simulink model "Model"  (R2023a)
settings: Solver=ode3  StartTime=0.0  StopTime=2.0  FixedStep=0.0001  RelTol=1e-3
values from neighbouring files (symbols this model uses):
  J2 = 1.26e-3    (= 0.00126)    [system_init.m]
libraries: neural x24
(part 1 of 2)
settings Model: SimulationMode=accelerator  Creator=04  LastModifiedBy=23688
settings SolverCC: AlgebraicLoopSolver=TrustRegion
settings DataIOCC: ReturnWorkspaceOutputs=off
settings DebuggingCC: UnconnectedInputMsg=warning  UnconnectedOutputMsg=warning  UnconnectedLineMsg=warning
settings ModelReferenceCC: EnableRefExpFcnMdlSchedulingChecks=on
settings RTWCC: DLArmComputeVersion=19.05

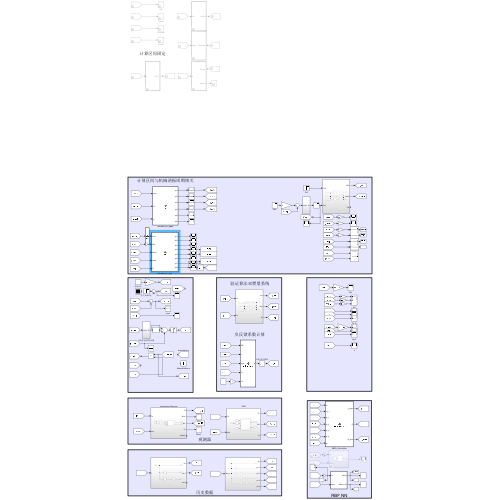
[thumbnail: Simulink's stored preview of the top-level diagram]
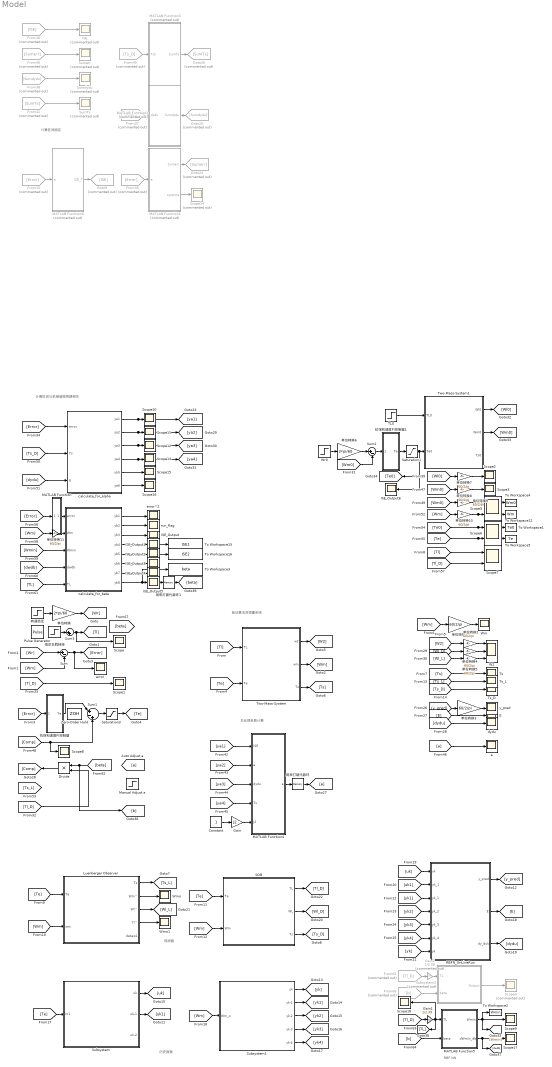
== system Model ==
  note: 观测器
  note: 历史数据
  note: 计算区间固定
  note: 计算区间与机械谐振周期相关
  note: 验证算法双惯量系统
  note: 负反馈系数计算
  note: RBF NN
  " Luenberger Observer" : Subsystem
  Constant : Constant
  Divide : Product  Inputs=**
  E : Scope
  From15 : From  Commented=on  GotoTag=Error
  From16 : From  Commented=on  GotoTag=ISE
  From35 : From  Commented=on  GotoTag=Error
  From36 : From  Commented=on  GotoTag=Sumerr
  From37 : From  Commented=on  GotoTag=dydu
  From38 : From  Commented=on  GotoTag=Sumdydu
  From40 : From  Commented=on  GotoTag=Ts_D
  From41 : From  Commented=on  GotoTag=SumTs
  From65 : From  Commented=on  GotoTag=Tl_D
  From66 : From  Commented=on  GotoTag=b
  Gain : Gain  Gain=J2
  Gain1 : Gain  Gain=1/2.39
  Gain2 : Gain  Commented=on  Gain=1/2.39
  Goto24 : Goto  Commented=on  GotoTag=Sumerr
  Goto25 : Goto  Commented=on  GotoTag=Sumdydu
  Goto26 : Goto  Commented=on  GotoTag=SumTs
  Goto9 : Goto  Commented=on  GotoTag=ISE
  ISE : Scope  Commented=on
  ISE_Output{,1..6} (7 alike) : Scope
  MATLAB Function : MATLAB Function  TreatAsAtomicUnit=on
  MATLAB Function1 : MATLAB Function  Commented=on  TreatAsAtomicUnit=on
  MATLAB Function2 : MATLAB Function  Commented=on  TreatAsAtomicUnit=on
  MATLAB Function3 : MATLAB Function  Commented=on  TreatAsAtomicUnit=on
  MATLAB Function4 : MATLAB Function  TreatAsAtomicUnit=on
  MATLAB Function5 : MATLAB Function  TreatAsAtomicUnit=on
  MATLAB Function6 : MATLAB Function  Commented=on  TreatAsAtomicUnit=on
  Manual Adjust a : Step  Time=0.1  After=0.0  SampleTime=0
  Pulse Generator : DiscretePulseGenerator  PulseType=Time based  Amplitude=2.39*0.7  Period=1  PulseWidth=50  PhaseDelay=1
  RBFN_OnLineRun : MATLAB Function  TreatAsAtomicUnit=on
  SOB : Subsystem
  Saturation1 : Saturate  UpperLimit=2.39*3  LowerLimit=-2.39*3
  Saturation3 : Saturate  UpperLimit=2.39*3  LowerLimit=-2.39*3
  Scope{,1..3,8..13,15..18} (14 alike) : Scope
  Scope14 : Scope  Commented=on
  Scope4 : Scope  Commented=on
  Scope5 : Scope  NumInputPorts=2
  Scope6 : Scope  NumInputPorts=2
  Scope7 : Scope  NumInputPorts=2
  Subsystem : Subsystem
  Subsystem1 : Subsystem
  Subsystem2 : Subsystem  Commented=on
  Sum : Sum  Inputs=|+-
  Sum1 : Sum  Inputs=|+-+
  Sum2 : Sum  Inputs=|+-
  Sum3 : Sum  Inputs=|++
  SumTs : Scope  Commented=on
  Sumdydu : Scope  Commented=on
  Sumerr : Scope  Commented=on
  TL0 : Step  After=2.39*0.5  SampleTime=0
  To Workspace1 : ToWorkspace  VariableName=Te0  SampleTime=-1
  To Workspace12 : ToWorkspace  VariableName=Wm  SampleTime=-1
  To Workspace15 : ToWorkspace  VariableName=ISE1  SampleTime=-1
  To Workspace16 : ToWorkspace  VariableName=ISE2  SampleTime=-1
  To Workspace2 : ToWorkspace  VariableName=Wmin  SampleTime=-1
  To Workspace3 : ToWorkspace  VariableName=beta  SampleTime=-1
  To Workspace4 : ToWorkspace  VariableName=Wm0  SampleTime=-1
  To Workspace5 : ToWorkspace  VariableName=Te  SampleTime=-1
  Ts : Scope
  Ts_D : Scope
  Ts_L : Scope
  Two-Mass-System : Subsystem
  Two-Mass-System1 : Subsystem
  W2 : Scope  NumInputPorts=3
  Wm : Scope
  Wmo : Scope
  Wmo1 : Scope
  Wr0 : Step  Time=0.1  After=1000  SampleTime=0
  Zero-Order Hold : ZeroOrderHold  SampleTime=0.0005
  a : Scope
  calculate_for_alpha : MATLAB Function  TreatAsAtomicUnit=on
  calculate_for_beta : MATLAB Function  TreatAsAtomicUnit=on
  dydu : Scope
  error : Scope
  error^2 : Scope
  run_flag : Scope
  y_pred : Scope
  单位转换 : Gain  Gain=2*pi/60
  单位转换{1..5,7..11} (10 alike) : Gain  Gain=60/2/pi
  单位转换6 : Gain  Gain=2*pi/60
  恒定负载转矩 : Step  After=2.39*0.5  SampleTime=0
  抗饱和速度PI控制器 : Subsystem
  抗饱和速度PI控制器1 : Subsystem
  用来打破代数环 : Memory  InheritSampleTime=on
  用来打破代数环1 : Memory  InheritSampleTime=on
  转速给定 : Step  Time=0.1  After=1000  SampleTime=0
  wires:
  [Tl] -> Two-Mass-System/1(TL)
  Two-Mass-System/2(wm) -> [Wm]
  [Wr] -> Sum/1
  [Wm] -> Sum/2
  Sum/1 -> error/1, [Error]
  [Error] -> 抗饱和速度PI控制器/1(error)
  Two-Mass-System/1(w2) -> [W2]
  Two-Mass-System/3(Ts) -> [Ts]
  [Ts] -> Ts/1
  单位转换/1 -> [Wr]
  [Wm] -> 单位转换1/1
  [Te] -> " Luenberger Observer"/1(Te)
  [Wm] -> " Luenberger Observer"/2(wm)
  [Te] -> SOB/1(Te)
  [Wm] -> SOB/2(Wm)
  " Luenberger Observer"/1(Ts) -> [Ts_L]
  SOB/3(Ts) -> [Ts_D]
  [Ts_L] -> Ts_L/1
  [Ts_D] -> Ts_D/1
  [W2] -> 单位转换2/1
  单位转换2/1 -> W2/1
  [Te] -> Subsystem/1(In1)
  Subsystem/1(uk) -> [uk]
  Subsystem/2(uk-1) -> [uk1]
  Subsystem1/1(yk) -> [yk]
  Subsystem1/2(yk-1) -> [yk1]
  Subsystem1/3(yk-2) -> [yk2]
  Subsystem1/4(yk-3) -> [yk3]
  Subsystem1/5(yk-4) -> [yk4]
  [uk] -> RBFN_OnLineRun/1(uk)
  [uk1] -> RBFN_OnLineRun/2(uk_1)
  [yk] -> RBFN_OnLineRun/7(yk)
  [yk1] -> RBFN_OnLineRun/3(yk_1)
  [yk2] -> RBFN_OnLineRun/4(yk_2)
  [yk3] -> RBFN_OnLineRun/5(yk_3)
  [yk4] -> RBFN_OnLineRun/6(yk_4)
  RBFN_OnLineRun/1(y_pred) -> [y_pred]
  RBFN_OnLineRun/2(E) -> [E]
  [E] -> E/1
  [dydu] -> dydu/1
  SOB/2(WL) -> [Wl_D]
  " Luenberger Observer"/3(Wl^) -> [Wl_L]
  单位转换4/1 -> W2/2
  [Wl_D] -> 单位转换4/1
  单位转换5/1 -> W2/3
  [Wl_L] -> 单位转换5/1
  单位转换1/1 -> Wm/1
  From35/1 -> MATLAB Function1/1(e)
  MATLAB Function1/1(Sumerr) -> Goto24/1
  From16/1 -> ISE/1
  From36/1 -> Sumerr/1
  From37/1 -> MATLAB Function2/1(dydu)
  MATLAB Function2/1(Sumdydu) -> Goto25/1
  From38/1 -> Sumdydu/1
  From40/1 -> MATLAB Function3/1(Tsk)
  MATLAB Function3/1(SumTs) -> Goto26/1
  From41/1 -> SumTs/1
  [ya1] -> MATLAB Function4/1(ISE)
  [ya2] -> MATLAB Function4/2(e)
  [ya3] -> MATLAB Function4/3(dydu)
  [ya4] -> MATLAB Function4/4(Ts)
  [a] -> a/1
  Divide/1 -> [Comp]
  [Te] -> Two-Mass-System/2(Te)
  MATLAB Function6/1(ISE_T) -> Goto9/1
  From15/1 -> MATLAB Function6/1(e)
  Gain/1 -> MATLAB Function4/5(J2)
  Constant/1 -> Gain/1
  SOB/1(TL) -> [Tl_D]
  [Tl_D] -> Scope1/1
  calculate_for_alpha/1(ya1) -> Scope10/1, [ya1]
  calculate_for_alpha/2(ya2) -> Scope11/1, [ya2]
  [Ts_D] -> calculate_for_alpha/2(Ts)
  calculate_for_alpha/3(ya3) -> [ya3], Scope12/1
  [dydu] -> calculate_for_alpha/3(g)
  calculate_for_alpha/4(ya4) -> [ya4], Scope13/1
  MATLAB Function4/1(a) -> 用来打破代数环/1
  RBFN_OnLineRun/3(dy_duk) -> [dydu]
  用来打破代数环/1 -> [a]
  MATLAB Function1/2(systime) -> Scope14/1
  calculate_for_alpha/5(ya5) -> Scope15/1
  calculate_for_alpha/6(ya6) -> Scope16/1
  Saturation3/1 -> [Te]
  " Luenberger Observer"/2(Wm^) -> Wmo/1
  转速给定/1 -> 单位转换/1
  [y_pred] -> 单位转换3/1
  单位转换3/1 -> y_pred/1
  [Wm] -> Subsystem1/1(Wm_o)
  [Error] -> calculate_for_alpha/1(error)
  Sum1/1 -> Saturation3/1
  Sum3/1 -> Scope/1, [Tl]
  calculate_for_beta/1(yb1) -> error^2/1
  calculate_for_beta/2(yb2) -> run_flag/1
  calculate_for_beta/3(yb3) -> ISE_Output/1
  calculate_for_beta/6(yb6) -> ISE_Output3/1
  calculate_for_beta/7(yb7) -> ISE_Output4/1
  [Tl_D] -> Divide/2
  [Error] -> MATLAB Function/1(error)
  抗饱和速度PI控制器/1(Te) -> Sum1/1
  [Comp] -> Scope8/1, Sum1/3
  " Luenberger Observer"/4(Tl^) -> Wmo1/1
  恒定负载转矩/1 -> Sum3/1
  抗饱和速度PI控制器1/1(Te) -> Saturation1/1
  Saturation1/1 -> ISE_Output6/1, [Te0], Two-Mass-System1/2(Te0)
  Wr0/1 -> 单位转换6/1
  Two-Mass-System1/1(Wl0) -> [Wl0]
  Two-Mass-System1/2(Wm0) -> [Wm0]
  单位转换6/1 -> Sum2/1
  Sum2/1 -> 抗饱和速度PI控制器1/1(error)
  [Wm0] -> Sum2/2
  [Wl0] -> 单位转换7/1
  [Wm0] -> 单位转换8/1
  单位转换7/1 -> Scope2/1
  单位转换8/1 -> Scope3/1
  TL0/1 -> Two-Mass-System1/1(TL0)
  [Wm0] -> 单位转换9/1
  单位转换9/1 -> To Workspace4/1, Scope5/1
  单位转换10/1 -> To Workspace12/1, Scope5/2
  [Wm] -> 单位转换10/1
  [Te] -> To Workspace5/1, Scope6/2
  [Tl] -> Scope7/1
  [Tl_D] -> Scope7/2
  MATLAB Function/1(error_output) -> calculate_for_beta/1(error)
  From65/1 -> Gain2/1
  Gain2/1 -> Subsystem2/1(TL)
  From66/1 -> Subsystem2/2(beta)
  Subsystem2/1(Output) -> Scope4/1
  [b] -> MATLAB Function5/2(beta)
  Gain1/1 -> Scope18/1, [TL], MATLAB Function5/1(TL)
  [Tl_D] -> Gain1/1
  MATLAB Function5/1(Wmin) -> To Workspace2/1, [Wmin], Scope9/1
  MATLAB Function5/2(dWmin_db) -> [dwdb], Scope17/1
  calculate_for_beta/5(yb5) -> To Workspace16/1, ISE_Output2/1
  calculate_for_beta/4(yb4) -> To Workspace15/1, ISE_Output1/1
  单位转换11/1 -> calculate_for_beta/2(Wm)
  [Wm] -> 单位转换11/1
  [Wmin] -> calculate_for_beta/3(Wmin)
  [dwdb] -> calculate_for_beta/4(dwdb)
  calculate_for_beta/8(yb8) -> To Workspace3/1, 用来打破代数环1/1, ISE_Output5/1
  [TL] -> calculate_for_beta/5(TL)
  用来打破代数环1/1 -> [beta]
  [beta] -> [b], Divide/1
  [Te0] -> To Workspace1/1, Scope6/1

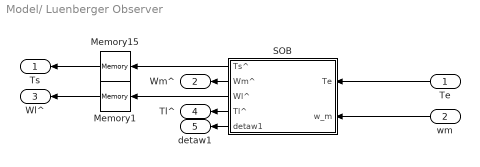
== system Model/ Luenberger Observer ==
  Te : Inport
  wm : Inport  Port=2
  Memory1 : Memory
  Memory15 : Memory
  SOB : Subsystem
  Ts : Outport
  Wm^ : Outport  Port=2
  Wl^ : Outport  Port=3
  Tl^ : Outport  Port=4
  detaw1 : Outport  Port=5
  wires:
  SOB/4(Tl^) -> Tl^/1
  SOB/1(Ts^) -> Memory15/1
  Memory15/1 -> Ts/1
  wm/1 -> SOB/2(w_m)
  SOB/2(Wm^) -> Wm^/1
  Te/1 -> SOB/1(Te)
  SOB/5(detaw1) -> detaw1/1
  Memory1/1 -> Wl^/1
  SOB/3(Wl^) -> Memory1/1

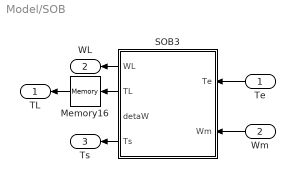
== system Model/SOB ==
  Te : Inport
  Wm : Inport  Port=2
  Memory16 : Memory
  SOB3 : Subsystem
  TL : Outport
  WL : Outport  Port=2
  Ts : Outport  Port=3
  wires:
  SOB3/1(WL) -> WL/1
  SOB3/4(Ts) -> Ts/1
  Wm/1 -> SOB3/2(Wm)
  Te/1 -> SOB3/1(Te)
  SOB3/2(TL) -> Memory16/1
  Memory16/1 -> TL/1

== system Model/Subsystem ==
  In1 : Inport
  Unit Delay : UnitDelay  SampleTime=-1  HasFrameUpgradeWarning=on
  Unit Delay1 : UnitDelay  SampleTime=-1  HasFrameUpgradeWarning=on
  Unit Delay2 : UnitDelay  SampleTime=-1  HasFrameUpgradeWarning=on
  uk : Outport
  uk-1 : Outport  Port=2
  uk-2 : Outport  Port=3
  wires:
  Unit Delay1/1 -> Unit Delay2/1
  Unit Delay/1 -> uk-1/1
  Unit Delay2/1 -> uk-2/1
  In1/1 -> Unit Delay1/1, Unit Delay/1, uk/1

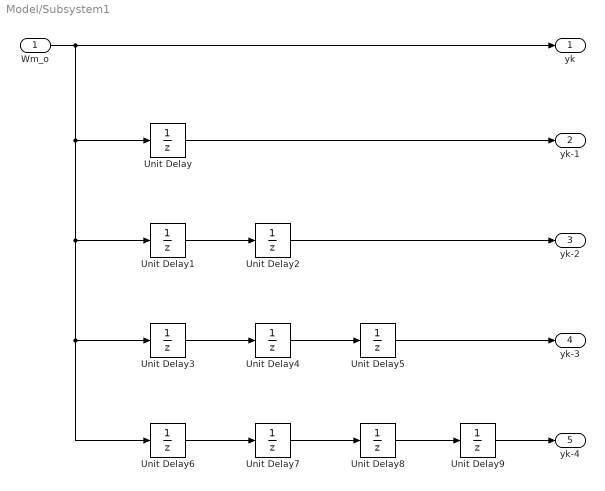
== system Model/Subsystem1 ==
  Wm_o : Inport
  Unit Delay{,1..9} (10 alike) : UnitDelay  SampleTime=-1  HasFrameUpgradeWarning=on
  yk : Outport
  yk-1 : Outport  Port=2
  yk-2 : Outport  Port=3
  yk-3 : Outport  Port=4
  yk-4 : Outport  Port=5
  wires:
  Unit Delay5/1 -> yk-3/1
  Unit Delay4/1 -> Unit Delay5/1
  Unit Delay2/1 -> yk-2/1
  Unit Delay8/1 -> Unit Delay9/1
  Unit Delay7/1 -> Unit Delay8/1
  Unit Delay6/1 -> Unit Delay7/1
  Unit Delay9/1 -> yk-4/1
  Unit Delay3/1 -> Unit Delay4/1
  Unit Delay/1 -> yk-1/1
  Wm_o/1 -> Unit Delay3/1, Unit Delay6/1, Unit Delay1/1, Unit Delay/1, yk/1
  Unit Delay1/1 -> Unit Delay2/1

== system Model/Subsystem2 ==
  TL : Inport
  beta : Inport  Port=2
  MATLAB Function7 : MATLAB Function  TreatAsAtomicUnit=on
  Radial Basis Network : Subsystem
      mask help: Radial Basis Network
      mask Display: e = 0.06;c1 = [120 150 230]/255;c2 = ([120 150 230]+0)/383;c3 = ([120 150 230]+128)/383;patch([0 1 1 0],[0 0 1 1],c1);patch([0 1 1 1-e 1-e 0+e],[0 0 1 1-e 0+e 0+e],c2);patch([0 0 1 1-e 0+e 0+e],[0 1 1 1-e 1-e 0+e],c3);plot([0 1 1 0 0],[0 0 1 1 0]);fprintf('NNET');port_label('input',1,' Input');port_label('output',1,'Output ');
  Output : Outport
  wires:
  MATLAB Function7/1(y) -> Radial Basis Network/1(Input)
  TL/1 -> MATLAB Function7/1(TL)
  beta/1 -> MATLAB Function7/2(beta)
  Radial Basis Network/1(Output) -> Output/1

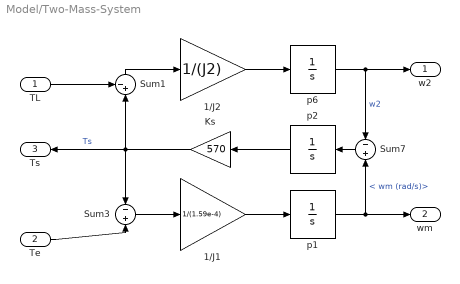
== system Model/Two-Mass-System ==
  TL : Inport
  Te : Inport  Port=2
  1/J1 : Gain  Gain=1/(1.59e-4)
  1/J2 : Gain  Gain=1/(J2)
  Ks : Gain  Gain=570
  Sum1 : Sum  Inputs=-+|
  Sum3 : Sum  Inputs=-+
  Sum7 : Sum  Inputs=-+
  p1 : TransferFcn  Denominator=[1 0]
  p2 : TransferFcn  Denominator=[1 0]
  p6 : TransferFcn  Denominator=[1 0]
  w2 : Outport
  wm : Outport  Port=2
  Ts : Outport  Port=3
  wires:
  Sum3/1 -> 1/J1/1
  1/J1/1 -> p1/1
  p1/1 -> wm/1, Sum7/2  "< wm (rad/s)>"
  p6/1 -> Sum7/1, w2/1  "w2"
  Sum7/1 -> p2/1
  Sum1/1 -> 1/J2/1
  Ks/1 -> Ts/1, Sum1/2, Sum3/1  "Ts"
  p2/1 -> Ks/1
  1/J2/1 -> p6/1
  TL/1 -> Sum1/1
  Te/1 -> Sum3/2

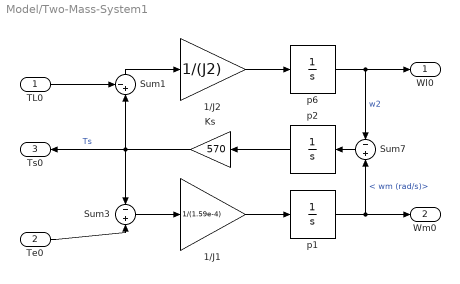
== system Model/Two-Mass-System1 ==
  TL0 : Inport
  Te0 : Inport  Port=2
  1/J1 : Gain  Gain=1/(1.59e-4)
  1/J2 : Gain  Gain=1/(J2)
  Ks : Gain  Gain=570
  Sum1 : Sum  Inputs=-+|
  Sum3 : Sum  Inputs=-+
  Sum7 : Sum  Inputs=-+
  p1 : TransferFcn  Denominator=[1 0]
  p2 : TransferFcn  Denominator=[1 0]
  p6 : TransferFcn  Denominator=[1 0]
  Wl0 : Outport
  Wm0 : Outport  Port=2
  Ts0 : Outport  Port=3
  wires:
  Sum3/1 -> 1/J1/1
  1/J1/1 -> p1/1
  p1/1 -> Wm0/1, Sum7/2  "< wm (rad/s)>"
  p6/1 -> Sum7/1, Wl0/1  "w2"
  Sum7/1 -> p2/1
  Sum1/1 -> 1/J2/1
  Ks/1 -> Ts0/1, Sum1/2, Sum3/1  "Ts"
  p2/1 -> Ks/1
  1/J2/1 -> p6/1
  TL0/1 -> Sum1/1
  Te0/1 -> Sum3/2

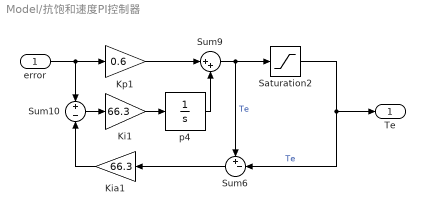
== system Model/抗饱和速度PI控制器 ==
  error : Inport
  Ki1 : Gain  Gain=66.3
  Kia1 : Gain  Gain=66.3
  Kp1 : Gain  Gain=0.6
  Saturation2 : Saturate  UpperLimit=2.39*3  LowerLimit=-2.39*3
  Sum10 : Sum  Inputs=+|-
  Sum6 : Sum  Inputs=+-|
  Sum9 : Sum  Inputs=|++
  p4 : TransferFcn  Denominator=[1 0]
  Te : Outport
  wires:
  Kia1/1 -> Sum10/2
  Sum6/1 -> Kia1/1
  Sum10/1 -> Ki1/1
  Kp1/1 -> Sum9/1
  Saturation2/1 -> Sum6/2, Te/1  "Te"
  Sum9/1 -> Sum6/1, Saturation2/1  "Te"
  p4/1 -> Sum9/2
  Ki1/1 -> p4/1
  error/1 -> Kp1/1, Sum10/1

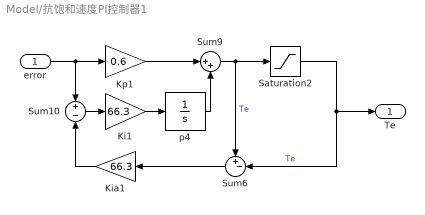
== system Model/抗饱和速度PI控制器1 ==
  error : Inport
  Ki1 : Gain  Gain=66.3
  Kia1 : Gain  Gain=66.3
  Kp1 : Gain  Gain=0.6
  Saturation2 : Saturate  UpperLimit=2.39*3  LowerLimit=-2.39*3
  Sum10 : Sum  Inputs=+|-
  Sum6 : Sum  Inputs=+-|
  Sum9 : Sum  Inputs=|++
  p4 : TransferFcn  Denominator=[1 0]
  Te : Outport
  wires:
  Kia1/1 -> Sum10/2
  Sum6/1 -> Kia1/1
  Sum10/1 -> Ki1/1
  Kp1/1 -> Sum9/1
  Saturation2/1 -> Sum6/2, Te/1  "Te"
  Sum9/1 -> Sum6/1, Saturation2/1  "Te"
  p4/1 -> Sum9/2
  Ki1/1 -> p4/1
  error/1 -> Kp1/1, Sum10/1

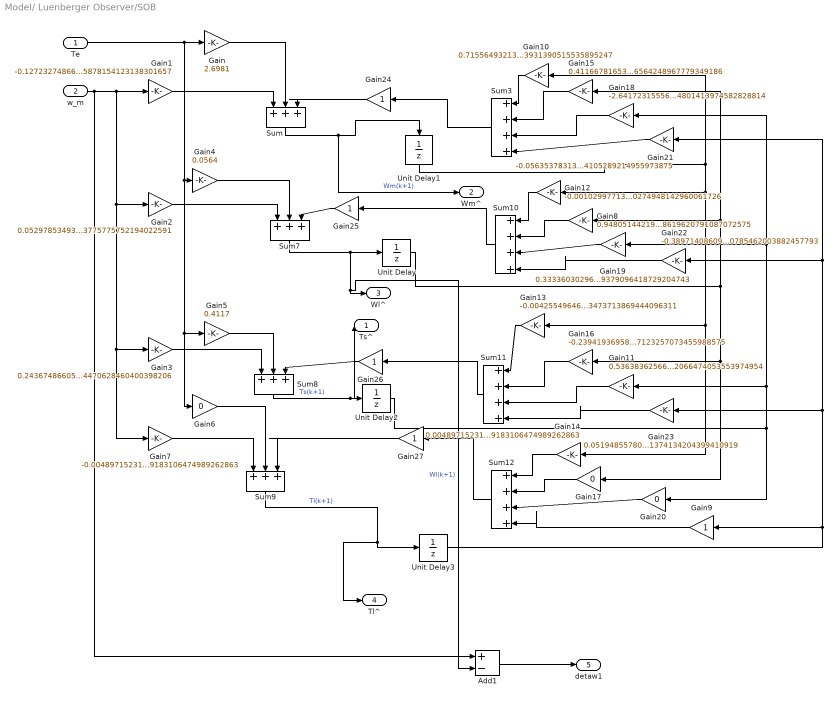
== system Model/ Luenberger Observer/SOB ==
  Te : Inport
  w_m : Inport  Port=2
  Add1 : Sum  Inputs=+-
  Gain : Gain  Gain=2.6981
  Gain1 : Gain  Gain=-0.12723274866755878154123138301657
  Gain10 : Gain  Gain=0.7155649321343931390515535895247
  Gain11 : Gain  Gain=0.53638362566622066474053553974954
  Gain12 : Gain  Gain=-0.0010299771306700274948142960061726
  Gain13 : Gain  Gain=-0.004255496467973473713869444096311
  Gain14 : Gain  Gain=0.0048971523131869183106474989262863
  Gain15 : Gain  Gain=0.41166781653316564248967779349186
  Gain16 : Gain  Gain=-0.23941936958917123257073455988575
  Gain17 : Gain  Gain=0
  Gain18 : Gain  Gain=-2.6417231555684801413974582828814
  Gain19 : Gain  Gain=0.33336030296459379096418729204743
  Gain2 : Gain  Gain=0.052978534931283775775752194022591
  Gain20 : Gain  Gain=0
  Gain21 : Gain  Gain=-0.056353783132214105289214955973875
  Gain22 : Gain  Gain=-0.38971408609680785462003882457793
  Gain23 : Gain  Gain=0.05194855780061374134204399410919
  Gain{9,24..27} (5 alike) : Gain
  Gain3 : Gain  Gain=0.24367486605714470628460400398206
  Gain4 : Gain  Gain=0.0564
  Gain5 : Gain  Gain=0.4117
  Gain6 : Gain  Gain=0
  Gain7 : Gain  Gain=-0.0048971523131869183106474989262863
  Gain8 : Gain  Gain=0.94805144219938619620791087072575
  Sum{,7..9} (4 alike) : Sum  Inputs=+++|
  Sum{3,10..12} (4 alike) : Sum  Inputs=++++|
  Unit Delay{,1..3} (4 alike) : UnitDelay  SampleTime=-1
  Ts^ : Outport
  Wm^ : Outport  Port=2
  Wl^ : Outport  Port=3
  Tl^ : Outport  Port=4
  detaw1 : Outport  Port=5
  wires:
  Te/1 -> Gain5/1, Gain6/1, Gain4/1, Gain/1
  Gain/1 -> Sum/2
  Gain1/1 -> Sum/1
  Gain4/1 -> Sum7/2
  Gain2/1 -> Sum7/1
  Gain5/1 -> Sum8/2
  Gain3/1 -> Sum8/1
  Gain6/1 -> Sum9/2
  Gain7/1 -> Sum9/1
  Sum/1 -> Unit Delay1/1, Wm^/1  "Wm(k+1)"
  Sum7/1 -> Add1/2, Wl^/1, Unit Delay/1  "Wl(k+1)"
  Sum8/1 -> Ts^/1, Unit Delay2/1  "Ts(k+1)"
  Sum9/1 -> Tl^/1, Unit Delay3/1  "Tl(k+1)"
  Sum12/1 -> Gain27/1
  Gain10/1 -> Sum3/1
  Gain11/1 -> Sum11/3
  Gain9/1 -> Sum12/4
  Gain12/1 -> Sum10/1
  Gain13/1 -> Sum11/1
  Gain14/1 -> Sum12/1
  Gain17/1 -> Sum12/2
  Gain19/1 -> Sum10/3
  Unit Delay1/1 -> Gain14/1, Gain13/1, Gain12/1, Gain10/1
  Unit Delay/1 -> Gain8/1, Gain15/1, Gain17/1, Gain16/1
  Unit Delay2/1 -> Gain11/1, Gain18/1, Gain19/1, Gain20/1
  Unit Delay3/1 -> Gain21/1, Gain22/1, Gain23/1, Gain9/1
  Gain25/1 -> Sum7/3
  Gain26/1 -> Sum8/3
  Sum3/1 -> Gain24/1
  Gain24/1 -> Sum/3
  Gain15/1 -> Sum3/2
  Gain18/1 -> Sum3/3
  Gain21/1 -> Sum3/4
  Sum10/1 -> Gain25/1
  Gain8/1 -> Sum10/2
  Sum11/1 -> Gain26/1
  Gain16/1 -> Sum11/2
  Gain23/1 -> Sum11/4
  Gain27/1 -> Sum9/3
  Gain20/1 -> Sum12/3
  Gain22/1 -> Sum10/4
  Add1/1 -> detaw1/1
  w_m/1 -> Add1/1, Gain3/1, Gain7/1, Gain2/1, Gain1/1

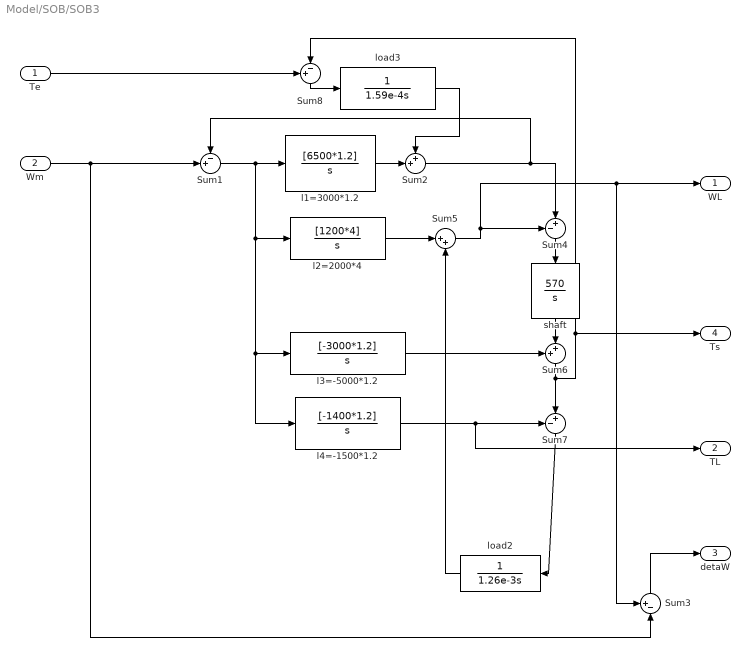
== system Model/SOB/SOB3 ==
  Te : Inport
  Wm : Inport  Port=2
  Sum1 : Sum  Inputs=-+|
  Sum2 : Sum  Inputs=++|
  Sum3 : Sum  Inputs=+-|
  Sum4 : Sum  Inputs=-+|
  Sum5 : Sum  Inputs=|++
  Sum6 : Sum  Inputs=++|
  Sum7 : Sum  Inputs=-+|
  Sum8 : Sum  Inputs=+-|
  l1=3000*1.2 : TransferFcn  Numerator=[6500*1.2]  Denominator=[1 0]
  l2=2000*4 : TransferFcn  Numerator=[1200*4]  Denominator=[1 0]
  l3=-5000*1.2 : TransferFcn  Numerator=[-3000*1.2]  Denominator=[1 0]
  l4=-1500*1.2 : TransferFcn  Numerator=[-1400*1.2]  Denominator=[1 0]
  load2 : TransferFcn  Denominator=[1.26e-3 0]
  load3 : TransferFcn  Denominator=[1.59e-4 0]
  shaft : TransferFcn  Numerator=[570]  Denominator=[1 0]
  WL : Outport  VectorParamsAs1DForOutWhenUnconnected=off
  TL : Outport  Port=2  VectorParamsAs1DForOutWhenUnconnected=off
  detaW : Outport  Port=3  VectorParamsAs1DForOutWhenUnconnected=off
  Ts : Outport  Port=4  VectorParamsAs1DForOutWhenUnconnected=off
  wires:
  Wm/1 -> Sum1/2, Sum3/2
  Te/1 -> Sum8/1
  load3/1 -> Sum2/1
  Sum8/1 -> load3/1
  load2/1 -> Sum5/2
  Sum7/1 -> load2/1
  Sum6/1 -> Sum7/2, Ts/1, Sum8/2
  l4=-1500*1.2/1 -> TL/1, Sum7/1
  shaft/1 -> Sum6/2
  l3=-5000*1.2/1 -> Sum6/1
  Sum4/1 -> shaft/1
  Sum5/1 -> WL/1, Sum3/1, Sum4/1
  l2=2000*4/1 -> Sum5/1
  Sum2/1 -> Sum4/2, Sum1/1
  l1=3000*1.2/1 -> Sum2/2
  Sum1/1 -> l4=-1500*1.2/1, l3=-5000*1.2/1, l2=2000*4/1, l1=3000*1.2/1
  Sum3/1 -> detaW/1

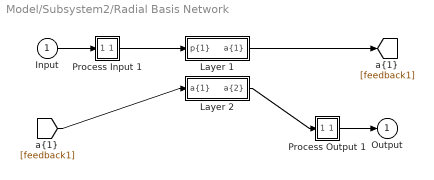
== system Model/Subsystem2/Radial Basis Network ==
  Input : Inport  PortDimensions=2
      mask Display: e = 0.06;c1 = [120 230 180]/255;c2 = ([120 230 180]+0)/(256+128);c3 = ([120 230 180]+128)/(256+128);patch([0 1 1 0],[0 0 1 1],c1);patch([0 1 1 1-e 1-e 0+e],[0 0 1 1-e 0+e 0+e],c2);patch([0 0 1 1-e 0+e 0+e],[0 1 1 1-e 1-e 0+e],c3);plot([0 1 1 0 0],[0 0 1 1 0]);
  Layer 1 : Subsystem
      mask Display: e = 0.06;c1 = [120 150 230]/255;c2 = ([120 150 230]+0)/383;c3 = ([120 150 230]+128)/383;patch([0 1 1 0],[0 0 1 1],c1);patch([0 1 1 1-e 1-e 0+e],[0 0 1 1-e 0+e 0+e],c2);patch([0 0 1 1-e 0+e 0+e],[0 1 1 1-e 1-e 0+e],c3);plot([0 1 1 0 0],[0 0 1 1 0]);
  Layer 2 : Subsystem
      mask Display: e = 0.06;c1 = [120 150 230]/255;c2 = ([120 150 230]+0)/383;c3 = ([120 150 230]+128)/383;patch([0 1 1 0],[0 0 1 1],c1);patch([0 1 1 1-e 1-e 0+e],[0 0 1 1-e 0+e 0+e],c2);patch([0 0 1 1-e 0+e 0+e],[0 1 1 1-e 1-e 0+e],c3);plot([0 1 1 0 0],[0 0 1 1 0]);
  Process Input 1 : Subsystem
      mask Display: e = 0.06;c1 = [120 150 230]/255;c2 = ([120 150 230]+0)/383;c3 = ([120 150 230]+128)/383;patch([0 1 1 0],[0 0 1 1],c1);patch([0 1 1 1-e 1-e 0+e],[0 0 1 1-e 0+e 0+e],c2);patch([0 0 1 1-e 0+e 0+e],[0 1 1 1-e 1-e 0+e],c3);plot([0 1 1 0 0],[0 0 1 1 0]);
  Process Output 1 : Subsystem
      mask Display: e = 0.06;c1 = [120 150 230]/255;c2 = ([120 150 230]+0)/383;c3 = ([120 150 230]+128)/383;patch([0 1 1 0],[0 0 1 1],c1);patch([0 1 1 1-e 1-e 0+e],[0 0 1 1-e 0+e 0+e],c2);patch([0 0 1 1-e 0+e 0+e],[0 1 1 1-e 1-e 0+e],c3);plot([0 1 1 0 0],[0 0 1 1 0]);
  Output : Outport  InitialOutput=0
      mask Display: e = 0.06;c1 = [120 230 180]/255;c2 = ([120 230 180]+0)/(256+128);c3 = ([120 230 180]+128)/(256+128);patch([0 1 1 0],[0 0 1 1],c1);patch([0 1 1 1-e 1-e 0+e],[0 0 1 1-e 0+e 0+e],c2);patch([0 0 1 1-e 0+e 0+e],[0 1 1 1-e 1-e 0+e],c3);plot([0 1 1 0 0],[0 0 1 1 0]);
  wires:
  Input/1 -> Process Input 1/1(x)
  Process Output 1/1(y) -> Output/1
  Process Input 1/1(p) -> Layer 1/1("p{1}")
  Layer 1/1("a{1}") -> [feedback1]
  [feedback1] -> Layer 2/1("a{1} ")
  Layer 2/1("a{2}") -> Process Output 1/1(a)

== system Model/Subsystem2/Radial Basis Network/Layer 1 ==
  "p{1}" : Inport  PortDimensions=2
      mask Display: e = 0.06;c1 = [120 230 180]/255;c2 = ([120 230 180]+0)/(256+128);c3 = ([120 230 180]+128)/(256+128);patch([0 1 1 0],[0 0 1 1],c1);patch([0 1 1 1-e 1-e 0+e],[0 0 1 1-e 0+e 0+e],c2);patch([0 0 1 1-e 0+e 0+e],[0 1 1 1-e 1-e 0+e],c3);plot([0 1 1 0 0],[0 0 1 1 0]);
  Delays 1 : Subsystem
      mask Display: e = 0.06;c1 = [120 150 230]/255;c2 = ([120 150 230]+0)/383;c3 = ([120 150 230]+128)/383;patch([0 1 1 0],[0 0 1 1],c1);patch([0 1 1 1-e 1-e 0+e],[0 0 1 1-e 0+e 0+e],c2);patch([0 0 1 1-e 0+e 0+e],[0 1 1 1-e 1-e 0+e],c3);plot([0 1 1 0 0],[0 0 1 1 0]);disp('0');
  "IW{1,1}" : Subsystem
      mask Display: e = 0.06;c1 = [120 150 230]/255;c2 = ([120 150 230]+0)/383;c3 = ([120 150 230]+128)/383;patch([0 1 1 0],[0 0 1 1],c1);patch([0 1 1 1-e 1-e 0+e],[0 0 1 1-e 0+e 0+e],c2);patch([0 0 1 1-e 0+e 0+e],[0 1 1 1-e 1-e 0+e],c3);plot([0 1 1 0 0],[0 0 1 1 0]);disp('W');
  "b{1}" : Constant  Value=[0.83255461115769768820626950400765053927898406982421875;0.83255461115769768820626950400765053927898406982421875;0.83255461115769768820626950400765053927898406982421875;0.83255461115769768820626950400765053927898406982421875;0.83255461115769768820626950400765053927898406982421875;0.83255461115769768820626950400765053927898406982421875;0.83255461115769768820626950400765053927898406982421875;0.83255461115769768820626950400765053927898406982421875;0.83255461115769768820626950400765053927898406982421875;0.83255461115769768820626950400765053927898406982421875;0.83255461115769768820626950400765053927898406982421875;0.83255461115769768820626950400765053927898406982421875;0.83255461115769768820626950400765053927898406982421875;0.83255461115769768820626950400765053927898406982421875;0.83255461115769768820626950400765053927898406982421875;0.83255461115769768820626950400765053927898406982421875;0.83255461115769768820626950400765053927898406982421875;0.83255461115769768820626950400765053927898406982421875;0.83255461115769768820626950400765053927898406982421875;0.83255461115769768820626950400765053927898406982421875;0.83255461115769768820626950400765053927898406982421875]
      mask Display: e = 0.06;c1 = [120 150 230]/255;c2 = ([120 150 230]+0)/383;c3 = ([120 150 230]+128)/383;patch([0 1 1 0],[0 0 1 1],c1);patch([0 1 1 1-e 1-e 0+e],[0 0 1 1-e 0+e 0+e],c2);patch([0 0 1 1-e 0+e 0+e],[0 1 1 1-e 1-e 0+e],c3);plot([0 1 1 0 0],[0 0 1 1 0]);disp('b');
  netprod : Product  InputSameDT=on  RndMeth=Zero  SaturateOnIntegerOverflow=on  OutDataTypeStr=Inherit: Same as first input
      mask Display: e = 0.06;c1 = [120 150 230]/255;c2 = ([120 150 230]+0)/383;c3 = ([120 150 230]+128)/383;patch([0 1 1 0],[0 0 1 1],c1);patch([0 1 1 1-e 1-e 0+e],[0 0 1 1-e 0+e 0+e],c2);patch([0 0 1 1-e 0+e 0+e],[0 1 1 1-e 1-e 0+e],c3);plot([0 1 1 0 0],[0 0 1 1 0]);disp('*');
  radbas : neural/Transfer Functions/radbas
  "a{1}" : Outport  InitialOutput=[0;0;0;0;0;0;0;0;0;0;0;0;0;0;0;0;0;0;0;0;0]
      mask Display: e = 0.06;c1 = [120 230 180]/255;c2 = ([120 230 180]+0)/(256+128);c3 = ([120 230 180]+128)/(256+128);patch([0 1 1 0],[0 0 1 1],c1);patch([0 1 1 1-e 1-e 0+e],[0 0 1 1-e 0+e 0+e],c2);patch([0 0 1 1-e 0+e 0+e],[0 1 1 1-e 1-e 0+e],c3);plot([0 1 1 0 0],[0 0 1 1 0]);
  wires:
  "p{1}"/1 -> Delays 1/1("p{1}")
  Delays 1/1("pd{1,1}") -> "IW{1,1}"/1("pd{1,1}")
  "IW{1,1}"/1("iz{1,1}") -> netprod/1
  "b{1}"/1 -> netprod/2
  netprod/1 -> radbas/1
  radbas/1 -> "a{1}"/1

== system Model/Subsystem2/Radial Basis Network/Layer 2 ==
  "a{1} " : Inport  PortDimensions=21
      mask Display: e = 0.06;c1 = [120 230 180]/255;c2 = ([120 230 180]+0)/(256+128);c3 = ([120 230 180]+128)/(256+128);patch([0 1 1 0],[0 0 1 1],c1);patch([0 1 1 1-e 1-e 0+e],[0 0 1 1-e 0+e 0+e],c2);patch([0 0 1 1-e 0+e 0+e],[0 1 1 1-e 1-e 0+e],c3);plot([0 1 1 0 0],[0 0 1 1 0]);
  Delays 1 : Subsystem
      mask Display: e = 0.06;c1 = [120 150 230]/255;c2 = ([120 150 230]+0)/383;c3 = ([120 150 230]+128)/383;patch([0 1 1 0],[0 0 1 1],c1);patch([0 1 1 1-e 1-e 0+e],[0 0 1 1-e 0+e 0+e],c2);patch([0 0 1 1-e 0+e 0+e],[0 1 1 1-e 1-e 0+e],c3);plot([0 1 1 0 0],[0 0 1 1 0]);disp('0');
  "LW{2,1}" : Subsystem
      mask Display: e = 0.06;c1 = [120 150 230]/255;c2 = ([120 150 230]+0)/383;c3 = ([120 150 230]+128)/383;patch([0 1 1 0],[0 0 1 1],c1);patch([0 1 1 1-e 1-e 0+e],[0 0 1 1-e 0+e 0+e],c2);patch([0 0 1 1-e 0+e 0+e],[0 1 1 1-e 1-e 0+e],c3);plot([0 1 1 0 0],[0 0 1 1 0]);disp('W');
  "b{2}" : Constant  Value=987.549222597197285722359083592891693115234375
      mask Display: e = 0.06;c1 = [120 150 230]/255;c2 = ([120 150 230]+0)/383;c3 = ([120 150 230]+128)/383;patch([0 1 1 0],[0 0 1 1],c1);patch([0 1 1 1-e 1-e 0+e],[0 0 1 1-e 0+e 0+e],c2);patch([0 0 1 1-e 0+e 0+e],[0 1 1 1-e 1-e 0+e],c3);plot([0 1 1 0 0],[0 0 1 1 0]);disp('b');
  netsum : Sum  Inputs=2  InputSameDT=on  SaturateOnIntegerOverflow=on  OutDataTypeStr=Inherit: Same as first input
      mask Display: e = 0.06;c1 = [120 150 230]/255;c2 = ([120 150 230]+0)/383;c3 = ([120 150 230]+128)/383;patch([0 1 1 0],[0 0 1 1],c1);patch([0 1 1 1-e 1-e 0+e],[0 0 1 1-e 0+e 0+e],c2);patch([0 0 1 1-e 0+e 0+e],[0 1 1 1-e 1-e 0+e],c3);plot([0 1 1 0 0],[0 0 1 1 0]);disp('+');
  purelin : neural/Transfer Functions/purelin
  "a{2}" : Outport  InitialOutput=0
      mask Display: e = 0.06;c1 = [120 230 180]/255;c2 = ([120 230 180]+0)/(256+128);c3 = ([120 230 180]+128)/(256+128);patch([0 1 1 0],[0 0 1 1],c1);patch([0 1 1 1-e 1-e 0+e],[0 0 1 1-e 0+e 0+e],c2);patch([0 0 1 1-e 0+e 0+e],[0 1 1 1-e 1-e 0+e],c3);plot([0 1 1 0 0],[0 0 1 1 0]);
  wires:
  "a{1} "/1 -> Delays 1/1("p{2}")
  Delays 1/1("pd{2,1}") -> "LW{2,1}"/1("ad{2,1}")
  "LW{2,1}"/1("lz{2,1}") -> netsum/1
  "b{2}"/1 -> netsum/2
  netsum/1 -> purelin/1
  purelin/1 -> "a{2}"/1

== system Model/Subsystem2/Radial Basis Network/Process Input 1 ==
  x : Inport  PortDimensions=2
      mask Display: e = 0.06;c1 = [120 230 180]/255;c2 = ([120 230 180]+0)/(256+128);c3 = ([120 230 180]+128)/(256+128);patch([0 1 1 0],[0 0 1 1],c1);patch([0 1 1 1-e 1-e 0+e],[0 0 1 1-e 0+e 0+e],c2);patch([0 0 1 1-e 0+e 0+e],[0 1 1 1-e 1-e 0+e],c3);plot([0 1 1 0 0],[0 0 1 1 0]);
  p : Outport  PortDimensions=2
      mask Display: e = 0.06;c1 = [120 230 180]/255;c2 = ([120 230 180]+0)/(256+128);c3 = ([120 230 180]+128)/(256+128);patch([0 1 1 0],[0 0 1 1],c1);patch([0 1 1 1-e 1-e 0+e],[0 0 1 1-e 0+e 0+e],c2);patch([0 0 1 1-e 0+e 0+e],[0 1 1 1-e 1-e 0+e],c3);plot([0 1 1 0 0],[0 0 1 1 0]);
  wires:
  x/1 -> p/1

== system Model/Subsystem2/Radial Basis Network/Process Output 1 ==
  a : Inport  PortDimensions=1
      mask Display: e = 0.06;c1 = [120 230 180]/255;c2 = ([120 230 180]+0)/(256+128);c3 = ([120 230 180]+128)/(256+128);patch([0 1 1 0],[0 0 1 1],c1);patch([0 1 1 1-e 1-e 0+e],[0 0 1 1-e 0+e 0+e],c2);patch([0 0 1 1-e 0+e 0+e],[0 1 1 1-e 1-e 0+e],c3);plot([0 1 1 0 0],[0 0 1 1 0]);
  y : Outport  PortDimensions=1
      mask Display: e = 0.06;c1 = [120 230 180]/255;c2 = ([120 230 180]+0)/(256+128);c3 = ([120 230 180]+128)/(256+128);patch([0 1 1 0],[0 0 1 1],c1);patch([0 1 1 1-e 1-e 0+e],[0 0 1 1-e 0+e 0+e],c2);patch([0 0 1 1-e 0+e 0+e],[0 1 1 1-e 1-e 0+e],c3);plot([0 1 1 0 0],[0 0 1 1 0]);
  wires:
  a/1 -> y/1

== system Model/Subsystem2/Radial Basis Network/Layer 1/Delays 1 ==
  "p{1}" : Inport  PortDimensions=2
      mask Display: e = 0.06;c1 = [120 230 180]/255;c2 = ([120 230 180]+0)/(256+128);c3 = ([120 230 180]+128)/(256+128);patch([0 1 1 0],[0 0 1 1],c1);patch([0 1 1 1-e 1-e 0+e],[0 0 1 1-e 0+e 0+e],c2);patch([0 0 1 1-e 0+e 0+e],[0 1 1 1-e 1-e 0+e],c3);plot([0 1 1 0 0],[0 0 1 1 0]);
  mux : Mux  Inputs=1
      mask Display: e = 0.06;c1 = [120 150 230]/255;c2 = ([120 150 230]+0)/383;c3 = ([120 150 230]+128)/383;patch([0 1 1 0],[0 0 1 1],c1);patch([0 1 1 1-e 1-e 0+e],[0 0 1 1-e 0+e 0+e],c2);patch([0 0 1 1-e 0+e 0+e],[0 1 1 1-e 1-e 0+e],c3);plot([0 1 1 0 0],[0 0 1 1 0]);disp('Mux')
  "pd{1,1}" : Outport
      mask Display: e = 0.06;c1 = [120 230 180]/255;c2 = ([120 230 180]+0)/(256+128);c3 = ([120 230 180]+128)/(256+128);patch([0 1 1 0],[0 0 1 1],c1);patch([0 1 1 1-e 1-e 0+e],[0 0 1 1-e 0+e 0+e],c2);patch([0 0 1 1-e 0+e 0+e],[0 1 1 1-e 1-e 0+e],c3);plot([0 1 1 0 0],[0 0 1 1 0]);
  wires:
  "p{1}"/1 -> mux/1
  mux/1 -> "pd{1,1}"/1

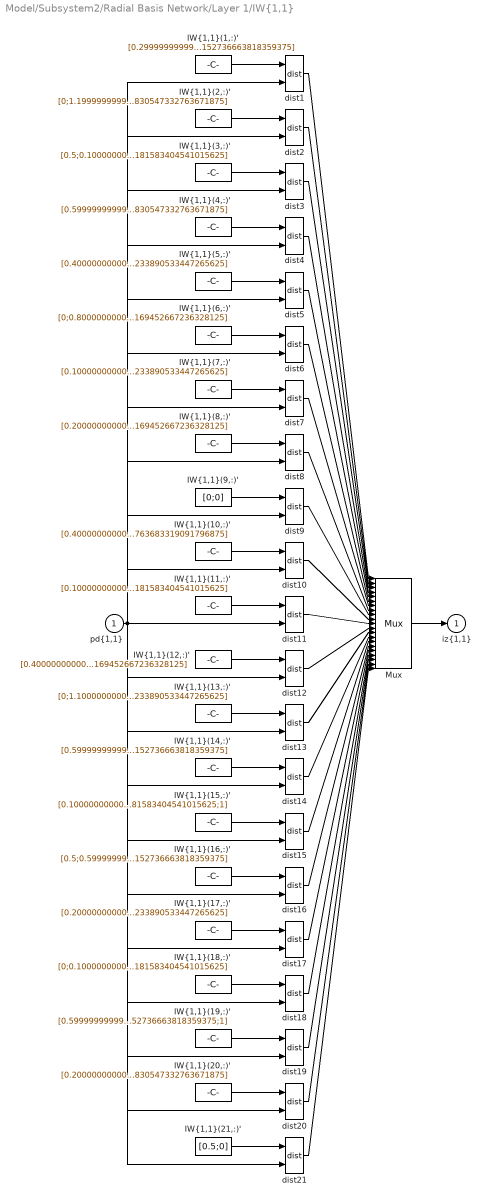
== system Model/Subsystem2/Radial Basis Network/Layer 1/IW{1,1} ==
  "pd{1,1}" : Inport  PortDimensions=2
      mask Display: e = 0.06;c1 = [120 230 180]/255;c2 = ([120 230 180]+0)/(256+128);c3 = ([120 230 180]+128)/(256+128);patch([0 1 1 0],[0 0 1 1],c1);patch([0 1 1 1-e 1-e 0+e],[0 0 1 1-e 0+e 0+e],c2);patch([0 0 1 1-e 0+e 0+e],[0 1 1 1-e 1-e 0+e],c3);plot([0 1 1 0 0],[0 0 1 1 0]);
  "IW{1,1}(1,:)'" : Constant  Value=[0.299999999999999988897769753748434595763683319091796875;0.59999999999999997779553950749686919152736663818359375]
      mask Display: e = 0.06;c1 = [120 150 230]/255;c2 = ([120 150 230]+0)/383;c3 = ([120 150 230]+128)/383;patch([0 1 1 0],[0 0 1 1],c1);patch([0 1 1 1-e 1-e 0+e],[0 0 1 1-e 0+e 0+e],c2);patch([0 0 1 1-e 0+e 0+e],[0 1 1 1-e 1-e 0+e],c3);plot([0 1 1 0 0],[0 0 1 1 0]);disp('Weights');
  "IW{1,1}(10,:)'" : Constant  Value=[0.40000000000000002220446049250313080847263336181640625;0.299999999999999988897769753748434595763683319091796875]
      mask Display: e = 0.06;c1 = [120 150 230]/255;c2 = ([120 150 230]+0)/383;c3 = ([120 150 230]+128)/383;patch([0 1 1 0],[0 0 1 1],c1);patch([0 1 1 1-e 1-e 0+e],[0 0 1 1-e 0+e 0+e],c2);patch([0 0 1 1-e 0+e 0+e],[0 1 1 1-e 1-e 0+e],c3);plot([0 1 1 0 0],[0 0 1 1 0]);disp('Weights');
  "IW{1,1}(11,:)'" : Constant  Value=[0.1000000000000000055511151231257827021181583404541015625;0.1000000000000000055511151231257827021181583404541015625]
      mask Display: e = 0.06;c1 = [120 150 230]/255;c2 = ([120 150 230]+0)/383;c3 = ([120 150 230]+128)/383;patch([0 1 1 0],[0 0 1 1],c1);patch([0 1 1 1-e 1-e 0+e],[0 0 1 1-e 0+e 0+e],c2);patch([0 0 1 1-e 0+e 0+e],[0 1 1 1-e 1-e 0+e],c3);plot([0 1 1 0 0],[0 0 1 1 0]);disp('Weights');
  "IW{1,1}(12,:)'" : Constant  Value=[0.40000000000000002220446049250313080847263336181640625;0.8000000000000000444089209850062616169452667236328125]
      mask Display: e = 0.06;c1 = [120 150 230]/255;c2 = ([120 150 230]+0)/383;c3 = ([120 150 230]+128)/383;patch([0 1 1 0],[0 0 1 1],c1);patch([0 1 1 1-e 1-e 0+e],[0 0 1 1-e 0+e 0+e],c2);patch([0 0 1 1-e 0+e 0+e],[0 1 1 1-e 1-e 0+e],c3);plot([0 1 1 0 0],[0 0 1 1 0]);disp('Weights');
  "IW{1,1}(13,:)'" : Constant  Value=[0;1.100000000000000088817841970012523233890533447265625]
      mask Display: e = 0.06;c1 = [120 150 230]/255;c2 = ([120 150 230]+0)/383;c3 = ([120 150 230]+128)/383;patch([0 1 1 0],[0 0 1 1],c1);patch([0 1 1 1-e 1-e 0+e],[0 0 1 1-e 0+e 0+e],c2);patch([0 0 1 1-e 0+e 0+e],[0 1 1 1-e 1-e 0+e],c3);plot([0 1 1 0 0],[0 0 1 1 0]);disp('Weights');
  "IW{1,1}(14,:)'" : Constant  Value=[0.59999999999999997779553950749686919152736663818359375;0.59999999999999997779553950749686919152736663818359375]
      mask Display: e = 0.06;c1 = [120 150 230]/255;c2 = ([120 150 230]+0)/383;c3 = ([120 150 230]+128)/383;patch([0 1 1 0],[0 0 1 1],c1);patch([0 1 1 1-e 1-e 0+e],[0 0 1 1-e 0+e 0+e],c2);patch([0 0 1 1-e 0+e 0+e],[0 1 1 1-e 1-e 0+e],c3);plot([0 1 1 0 0],[0 0 1 1 0]);disp('Weights');
  "IW{1,1}(15,:)'" : Constant  Value=[0.1000000000000000055511151231257827021181583404541015625;1]
      mask Display: e = 0.06;c1 = [120 150 230]/255;c2 = ([120 150 230]+0)/383;c3 = ([120 150 230]+128)/383;patch([0 1 1 0],[0 0 1 1],c1);patch([0 1 1 1-e 1-e 0+e],[0 0 1 1-e 0+e 0+e],c2);patch([0 0 1 1-e 0+e 0+e],[0 1 1 1-e 1-e 0+e],c3);plot([0 1 1 0 0],[0 0 1 1 0]);disp('Weights');
  "IW{1,1}(16,:)'" : Constant  Value=[0.5;0.59999999999999997779553950749686919152736663818359375]
      mask Display: e = 0.06;c1 = [120 150 230]/255;c2 = ([120 150 230]+0)/383;c3 = ([120 150 230]+128)/383;patch([0 1 1 0],[0 0 1 1],c1);patch([0 1 1 1-e 1-e 0+e],[0 0 1 1-e 0+e 0+e],c2);patch([0 0 1 1-e 0+e 0+e],[0 1 1 1-e 1-e 0+e],c3);plot([0 1 1 0 0],[0 0 1 1 0]);disp('Weights');
  "IW{1,1}(17,:)'" : Constant  Value=[0.200000000000000011102230246251565404236316680908203125;1.100000000000000088817841970012523233890533447265625]
      mask Display: e = 0.06;c1 = [120 150 230]/255;c2 = ([120 150 230]+0)/383;c3 = ([120 150 230]+128)/383;patch([0 1 1 0],[0 0 1 1],c1);patch([0 1 1 1-e 1-e 0+e],[0 0 1 1-e 0+e 0+e],c2);patch([0 0 1 1-e 0+e 0+e],[0 1 1 1-e 1-e 0+e],c3);plot([0 1 1 0 0],[0 0 1 1 0]);disp('Weights');
  "IW{1,1}(18,:)'" : Constant  Value=[0;0.1000000000000000055511151231257827021181583404541015625]
      mask Display: e = 0.06;c1 = [120 150 230]/255;c2 = ([120 150 230]+0)/383;c3 = ([120 150 230]+128)/383;patch([0 1 1 0],[0 0 1 1],c1);patch([0 1 1 1-e 1-e 0+e],[0 0 1 1-e 0+e 0+e],c2);patch([0 0 1 1-e 0+e 0+e],[0 1 1 1-e 1-e 0+e],c3);plot([0 1 1 0 0],[0 0 1 1 0]);disp('Weights');
  "IW{1,1}(19,:)'" : Constant  Value=[0.59999999999999997779553950749686919152736663818359375;1]
      mask Display: e = 0.06;c1 = [120 150 230]/255;c2 = ([120 150 230]+0)/383;c3 = ([120 150 230]+128)/383;patch([0 1 1 0],[0 0 1 1],c1);patch([0 1 1 1-e 1-e 0+e],[0 0 1 1-e 0+e 0+e],c2);patch([0 0 1 1-e 0+e 0+e],[0 1 1 1-e 1-e 0+e],c3);plot([0 1 1 0 0],[0 0 1 1 0]);disp('Weights');
  "IW{1,1}(2,:)'" : Constant  Value=[0;1.1999999999999999555910790149937383830547332763671875]
      mask Display: e = 0.06;c1 = [120 150 230]/255;c2 = ([120 150 230]+0)/383;c3 = ([120 150 230]+128)/383;patch([0 1 1 0],[0 0 1 1],c1);patch([0 1 1 1-e 1-e 0+e],[0 0 1 1-e 0+e 0+e],c2);patch([0 0 1 1-e 0+e 0+e],[0 1 1 1-e 1-e 0+e],c3);plot([0 1 1 0 0],[0 0 1 1 0]);disp('Weights');
  "IW{1,1}(20,:)'" : Constant  Value=[0.200000000000000011102230246251565404236316680908203125;0.6999999999999999555910790149937383830547332763671875]
      mask Display: e = 0.06;c1 = [120 150 230]/255;c2 = ([120 150 230]+0)/383;c3 = ([120 150 230]+128)/383;patch([0 1 1 0],[0 0 1 1],c1);patch([0 1 1 1-e 1-e 0+e],[0 0 1 1-e 0+e 0+e],c2);patch([0 0 1 1-e 0+e 0+e],[0 1 1 1-e 1-e 0+e],c3);plot([0 1 1 0 0],[0 0 1 1 0]);disp('Weights');
  "IW{1,1}(21,:)'" : Constant  Value=[0.5;0]
      mask Display: e = 0.06;c1 = [120 150 230]/255;c2 = ([120 150 230]+0)/383;c3 = ([120 150 230]+128)/383;patch([0 1 1 0],[0 0 1 1],c1);patch([0 1 1 1-e 1-e 0+e],[0 0 1 1-e 0+e 0+e],c2);patch([0 0 1 1-e 0+e 0+e],[0 1 1 1-e 1-e 0+e],c3);plot([0 1 1 0 0],[0 0 1 1 0]);disp('Weights');
  "IW{1,1}(3,:)'" : Constant  Value=[0.5;0.1000000000000000055511151231257827021181583404541015625]
      mask Display: e = 0.06;c1 = [120 150 230]/255;c2 = ([120 150 230]+0)/383;c3 = ([120 150 230]+128)/383;patch([0 1 1 0],[0 0 1 1],c1);patch([0 1 1 1-e 1-e 0+e],[0 0 1 1-e 0+e 0+e],c2);patch([0 0 1 1-e 0+e 0+e],[0 1 1 1-e 1-e 0+e],c3);plot([0 1 1 0 0],[0 0 1 1 0]);disp('Weights');
  "IW{1,1}(4,:)'" : Constant  Value=[0.59999999999999997779553950749686919152736663818359375;1.1999999999999999555910790149937383830547332763671875]
      mask Display: e = 0.06;c1 = [120 150 230]/255;c2 = ([120 150 230]+0)/383;c3 = ([120 150 230]+128)/383;patch([0 1 1 0],[0 0 1 1],c1);patch([0 1 1 1-e 1-e 0+e],[0 0 1 1-e 0+e 0+e],c2);patch([0 0 1 1-e 0+e 0+e],[0 1 1 1-e 1-e 0+e],c3);plot([0 1 1 0 0],[0 0 1 1 0]);disp('Weights');
  "IW{1,1}(5,:)'" : Constant  Value=[0.40000000000000002220446049250313080847263336181640625;1.100000000000000088817841970012523233890533447265625]
      mask Display: e = 0.06;c1 = [120 150 230]/255;c2 = ([120 150 230]+0)/383;c3 = ([120 150 230]+128)/383;patch([0 1 1 0],[0 0 1 1],c1);patch([0 1 1 1-e 1-e 0+e],[0 0 1 1-e 0+e 0+e],c2);patch([0 0 1 1-e 0+e 0+e],[0 1 1 1-e 1-e 0+e],c3);plot([0 1 1 0 0],[0 0 1 1 0]);disp('Weights');
  "IW{1,1}(6,:)'" : Constant  Value=[0;0.8000000000000000444089209850062616169452667236328125]
      mask Display: e = 0.06;c1 = [120 150 230]/255;c2 = ([120 150 230]+0)/383;c3 = ([120 150 230]+128)/383;patch([0 1 1 0],[0 0 1 1],c1);patch([0 1 1 1-e 1-e 0+e],[0 0 1 1-e 0+e 0+e],c2);patch([0 0 1 1-e 0+e 0+e],[0 1 1 1-e 1-e 0+e],c3);plot([0 1 1 0 0],[0 0 1 1 0]);disp('Weights');
  "IW{1,1}(7,:)'" : Constant  Value=[0.1000000000000000055511151231257827021181583404541015625;1.100000000000000088817841970012523233890533447265625]
      mask Display: e = 0.06;c1 = [120 150 230]/255;c2 = ([120 150 230]+0)/383;c3 = ([120 150 230]+128)/383;patch([0 1 1 0],[0 0 1 1],c1);patch([0 1 1 1-e 1-e 0+e],[0 0 1 1-e 0+e 0+e],c2);patch([0 0 1 1-e 0+e 0+e],[0 1 1 1-e 1-e 0+e],c3);plot([0 1 1 0 0],[0 0 1 1 0]);disp('Weights');
  "IW{1,1}(8,:)'" : Constant  Value=[0.200000000000000011102230246251565404236316680908203125;0.8000000000000000444089209850062616169452667236328125]
      mask Display: e = 0.06;c1 = [120 150 230]/255;c2 = ([120 150 230]+0)/383;c3 = ([120 150 230]+128)/383;patch([0 1 1 0],[0 0 1 1],c1);patch([0 1 1 1-e 1-e 0+e],[0 0 1 1-e 0+e 0+e],c2);patch([0 0 1 1-e 0+e 0+e],[0 1 1 1-e 1-e 0+e],c3);plot([0 1 1 0 0],[0 0 1 1 0]);disp('Weights');
  "IW{1,1}(9,:)'" : Constant  Value=[0;0]
      mask Display: e = 0.06;c1 = [120 150 230]/255;c2 = ([120 150 230]+0)/383;c3 = ([120 150 230]+128)/383;patch([0 1 1 0],[0 0 1 1],c1);patch([0 1 1 1-e 1-e 0+e],[0 0 1 1-e 0+e 0+e],c2);patch([0 0 1 1-e 0+e 0+e],[0 1 1 1-e 1-e 0+e],c3);plot([0 1 1 0 0],[0 0 1 1 0]);disp('Weights');
  Mux : Mux  Inputs=21
      mask Display: e = 0.06;c1 = [120 150 230]/255;c2 = ([120 150 230]+0)/383;c3 = ([120 150 230]+128)/383;patch([0 1 1 0],[0 0 1 1],c1);patch([0 1 1 1-e 1-e 0+e],[0 0 1 1-e 0+e 0+e],c2);patch([0 0 1 1-e 0+e 0+e],[0 1 1 1-e 1-e 0+e],c3);plot([0 1 1 0 0],[0 0 1 1 0]);disp('Mux');
  dist{1..21} (21 alike) : neural/Weight Functions/dist
  "iz{1,1}" : Outport
      mask Display: e = 0.06;c1 = [120 230 180]/255;c2 = ([120 230 180]+0)/(256+128);c3 = ([120 230 180]+128)/(256+128);patch([0 1 1 0],[0 0 1 1],c1);patch([0 1 1 1-e 1-e 0+e],[0 0 1 1-e 0+e 0+e],c2);patch([0 0 1 1-e 0+e 0+e],[0 1 1 1-e 1-e 0+e],c3);plot([0 1 1 0 0],[0 0 1 1 0]);
  wires:
  "IW{1,1}(1,:)'"/1 -> dist1/1
  "pd{1,1}"/1 -> dist1/2, dist2/2, dist3/2, dist4/2, dist5/2, dist6/2, dist7/2, dist8/2, dist9/2, dist10/2, dist11/2, dist12/2, dist13/2, dist14/2, dist15/2, dist16/2, dist17/2, dist18/2, dist19/2, dist20/2, dist21/2
  dist1/1 -> Mux/1
  "IW{1,1}(2,:)'"/1 -> dist2/1
  dist2/1 -> Mux/2
  "IW{1,1}(3,:)'"/1 -> dist3/1
  dist3/1 -> Mux/3
  "IW{1,1}(4,:)'"/1 -> dist4/1
  dist4/1 -> Mux/4
  "IW{1,1}(5,:)'"/1 -> dist5/1
  dist5/1 -> Mux/5
  "IW{1,1}(6,:)'"/1 -> dist6/1
  dist6/1 -> Mux/6
  "IW{1,1}(7,:)'"/1 -> dist7/1
  dist7/1 -> Mux/7
  "IW{1,1}(8,:)'"/1 -> dist8/1
  dist8/1 -> Mux/8
  "IW{1,1}(9,:)'"/1 -> dist9/1
  dist9/1 -> Mux/9
  "IW{1,1}(10,:)'"/1 -> dist10/1
  dist10/1 -> Mux/10
  "IW{1,1}(11,:)'"/1 -> dist11/1
  dist11/1 -> Mux/11
  "IW{1,1}(12,:)'"/1 -> dist12/1
  dist12/1 -> Mux/12
  "IW{1,1}(13,:)'"/1 -> dist13/1
  dist13/1 -> Mux/13
  "IW{1,1}(14,:)'"/1 -> dist14/1
  dist14/1 -> Mux/14
  "IW{1,1}(15,:)'"/1 -> dist15/1
  dist15/1 -> Mux/15
  "IW{1,1}(16,:)'"/1 -> dist16/1
  dist16/1 -> Mux/16
  "IW{1,1}(17,:)'"/1 -> dist17/1
  dist17/1 -> Mux/17
  "IW{1,1}(18,:)'"/1 -> dist18/1
  dist18/1 -> Mux/18
  "IW{1,1}(19,:)'"/1 -> dist19/1
  dist19/1 -> Mux/19
  "IW{1,1}(20,:)'"/1 -> dist20/1
  dist20/1 -> Mux/20
  "IW{1,1}(21,:)'"/1 -> dist21/1
  dist21/1 -> Mux/21
  Mux/1 -> "iz{1,1}"/1

== system Model/Subsystem2/Radial Basis Network/Layer 2/Delays 1 ==
  "p{2}" : Inport  PortDimensions=21
      mask Display: e = 0.06;c1 = [120 230 180]/255;c2 = ([120 230 180]+0)/(256+128);c3 = ([120 230 180]+128)/(256+128);patch([0 1 1 0],[0 0 1 1],c1);patch([0 1 1 1-e 1-e 0+e],[0 0 1 1-e 0+e 0+e],c2);patch([0 0 1 1-e 0+e 0+e],[0 1 1 1-e 1-e 0+e],c3);plot([0 1 1 0 0],[0 0 1 1 0]);
  mux : Mux  Inputs=1
      mask Display: e = 0.06;c1 = [120 150 230]/255;c2 = ([120 150 230]+0)/383;c3 = ([120 150 230]+128)/383;patch([0 1 1 0],[0 0 1 1],c1);patch([0 1 1 1-e 1-e 0+e],[0 0 1 1-e 0+e 0+e],c2);patch([0 0 1 1-e 0+e 0+e],[0 1 1 1-e 1-e 0+e],c3);plot([0 1 1 0 0],[0 0 1 1 0]);disp('Mux')
  "pd{2,1}" : Outport
      mask Display: e = 0.06;c1 = [120 230 180]/255;c2 = ([120 230 180]+0)/(256+128);c3 = ([120 230 180]+128)/(256+128);patch([0 1 1 0],[0 0 1 1],c1);patch([0 1 1 1-e 1-e 0+e],[0 0 1 1-e 0+e 0+e],c2);patch([0 0 1 1-e 0+e 0+e],[0 1 1 1-e 1-e 0+e],c3);plot([0 1 1 0 0],[0 0 1 1 0]);
  wires:
  "p{2}"/1 -> mux/1
  mux/1 -> "pd{2,1}"/1

== system Model/Subsystem2/Radial Basis Network/Layer 2/LW{2,1} ==
  "ad{2,1}" : Inport  PortDimensions=21
      mask Display: e = 0.06;c1 = [120 230 180]/255;c2 = ([120 230 180]+0)/(256+128);c3 = ([120 230 180]+128)/(256+128);patch([0 1 1 0],[0 0 1 1],c1);patch([0 1 1 1-e 1-e 0+e],[0 0 1 1-e 0+e 0+e],c2);patch([0 0 1 1-e 0+e 0+e],[0 1 1 1-e 1-e 0+e],c3);plot([0 1 1 0 0],[0 0 1 1 0]);
  "IW{2,1}(1,:)'" : Constant  Value=[-71051.84003394228057004511356353759765625;-38303.8677985831745900213718414306640625;-15672.521188910288401530124247074127197265625;140.845800400152683096166583709418773651123046875;9145.640846003223487059585750102996826171875;-686.6839494241231705018435604870319366455078125;147742.4062583116465248167514801025390625;95931.643959242268465459346771240234375;2290.10481683167336086626164615154266357421875;31679.23302361549940542317926883697509765625;-7411.74723482852641609497368335723876953125;10227.72728226036633714102208614349365234375;42907.297182661262922920286655426025390625;5223.9549026296981537598185241222381591796875;-171314.1919029368436895310878753662109375;-8160.011154380774314631707966327667236328125;-52059.173103113542310893535614013671875;1654.418151962109959640656597912311553955078125;-3625.6208196132574812509119510650634765625;15543.62662255172108416445553302764892578125;5808.5948080627631497918628156185150146484375]
      mask Display: e = 0.06;c1 = [120 150 230]/255;c2 = ([120 150 230]+0)/383;c3 = ([120 150 230]+128)/383;patch([0 1 1 0],[0 0 1 1],c1);patch([0 1 1 1-e 1-e 0+e],[0 0 1 1-e 0+e 0+e],c2);patch([0 0 1 1-e 0+e 0+e],[0 1 1 1-e 1-e 0+e],c3);plot([0 1 1 0 0],[0 0 1 1 0]);disp('weights');
  Mux : Mux  Inputs=1
      mask Display: e = 0.06;c1 = [120 150 230]/255;c2 = ([120 150 230]+0)/383;c3 = ([120 150 230]+128)/383;patch([0 1 1 0],[0 0 1 1],c1);patch([0 1 1 1-e 1-e 0+e],[0 0 1 1-e 0+e 0+e],c2);patch([0 0 1 1-e 0+e 0+e],[0 1 1 1-e 1-e 0+e],c3);plot([0 1 1 0 0],[0 0 1 1 0]);disp('Mux');
  dotprod1 : neural/Weight Functions/dotprod
  "lz{2,1}" : Outport
      mask Display: e = 0.06;c1 = [120 230 180]/255;c2 = ([120 230 180]+0)/(256+128);c3 = ([120 230 180]+128)/(256+128);patch([0 1 1 0],[0 0 1 1],c1);patch([0 1 1 1-e 1-e 0+e],[0 0 1 1-e 0+e 0+e],c2);patch([0 0 1 1-e 0+e 0+e],[0 1 1 1-e 1-e 0+e],c3);plot([0 1 1 0 0],[0 0 1 1 0]);
  wires:
  "IW{2,1}(1,:)'"/1 -> dotprod1/1
  "ad{2,1}"/1 -> dotprod1/2
  dotprod1/1 -> Mux/1
  Mux/1 -> "lz{2,1}"/1

== matlab function Model/calculate_for_beta ==
  settings: updateMethod=DISCRETE
  data: error input; yb1 output; yb2 output; yb3 output; yb4 output; yb5 output; yb6 output; yb7 output; Wm input; Wmin input; dwdb input; TL input; yb8 output
function [yb1, yb2, yb3, yb4, yb5, yb6, yb7, yb8]  = fcn(error,Wm,Wmin,dwdb,TL)

% 扰动检测、扰动ISE计算相关变量
persistent T time run_flag error_squa ISE_Output error_flag errorlast_flag err ISE1 ISE2 zero_count zeroerr_time zero_time Zero_Crossing_Time Time_Output Fd_ISE Fo_ISE Fd_time_low Fd_time_Up Fo_Flag Fd_Flag Fo_time_low Fo_time_Up

% beta计算相关变量
persistent Wm_Last beta_new beta_old Wr p

if isempty(T)
    T = 0.0001;                                        % 系统运行周期，s
    time = 0;                                          % 系统运行计时
    run_flag = 0;                                      % 状态标志位，初始化为0
    error_squa = 0;                                    % 误差平方值
    ISE_Output = 0;                                    % ISE输出值
    error_flag = 1;                                    % 当前时刻误差符号标志位
    errorlast_flag = 1;                                % 上一时刻误差符号标志位
    ISE1 = 0;
    ISE2 = 0;
    zero_count = 0;                                    % 过零点次数
    zeroerr_time = 0;                                  % 误差为0的时间
    zero_time = 0;                                     % 过零点计数时间窗口

    Zero_Crossing_Time = 0;                            % 相邻过零点时间间隔
    Time_Output = 0;                                   % 过零点时间间隔输出值

    Fo_ISE = 0.0001;                                   % 谐振ISE阈值
    Fd_ISE = 0.0144;                                   % 扰动ISE阈值
    
    Fd_time_low = 0.019;                               % 扰动时间下限，10%
    Fd_time_Up = 0.023;                                % 扰动时间上限，10%

    Fo_time_low = 0.00045;                             % 谐振时间下限，10%
    Fo_time_Up = 0.000055;                             % 谐振时间上限，10%

    Fo_Flag = 0;
    Fd_Flag = 0;
end

if isempty(Wm_Last)
    Wm_Last = 0;
    beta_new = 0;
    beta_old = 0;
    Wr = 1000;
    p = (5*5)/(3*3);                                 % 允许最大转速波动为10，1倍额定转矩（用的是标幺值）
end

err = error;

% 对当前时刻误差符号进行定义
if (err == 0)
    error_flag = 1;        % 误差为0
elseif (err > 0)
    error_flag = 2;        % 误差为正
elseif (err < 0)
    error_flag = 3;        % 误差为负
end


if (time > 0.8)  % 运行进入稳态再计算
  % 系统运行状态判断

  % 在状态0的前提下，误差信号的符号变化，发生过零，进入状态1
  if (run_flag == 0)
      if (errorlast_flag == 1 && error_flag == 2)                  % 0->+
          run_flag = 1;
      elseif (errorlast_flag == 1 && error_flag == 3)              % 0->-
          run_flag = 1;
      elseif (errorlast_flag == 3 && error_flag == 2)              % -->+
          run_flag = 1;
      elseif (errorlast_flag == 2 && error_flag == 3)              % +->-
          run_flag = 1;
      elseif (errorlast_flag == 3 && error_flag == 1)              % -->0
          run_flag = 1;
      elseif (errorlast_flag == 2 && error_flag == 1)              % +->0
          run_flag = 1;
      end
  end

  % 在状态1的前提下，误差信号的符号保持不变，进入状态2
  if (run_flag == 1)
      if ((errorlast_flag == 2 && error_flag == 2) || (errorlast_flag == 3 && error_flag == 3))
          run_flag = 2;
      end
  end

  % 在状态2的前提下，误差信号的符号变化，发生过零，进入状态3
  if (run_flag == 2)
      if (errorlast_flag == 2 && error_flag == 1)                  % +->0
          run_flag = 3;
      elseif (errorlast_flag == 3 && error_flag == 1)              % -->0
          run_flag = 3;
      elseif (errorlast_flag == 2 && error_flag == 3)              % +->-
          run_flag = 3;
      elseif (errorlast_flag == 3 && error_flag == 2)              % -->+
          run_flag = 3;
      end
  end

  % 每种状态对应的动作

  % 状态0，清空变量
  if (run_flag == 0)
      if (zero_count == 1)
          zeroerr_time = zeroerr_time + 1;
      end
  end
  
  % 状态1，清空变量，准备开始计算
  if (run_flag == 1)
      error_squa = 0;
      Zero_Crossing_Time = 0;
  end

  % 状态2，开始计算beta
  if (run_flag == 2)
      error_squa = error_squa + (err^2);
      Zero_Crossing_Time = Zero_Crossing_Time + T;

      % 判断是否属于转速下降阶段
      if (Wm - Wm_Last < 0 && abs(Wm - Wm_Last) > 0.1)                     % 0.3倍的阈值用0.01，0.5倍的阈值用0.1
          % 处于下降阶段，更新beta进行优化
          Error_max = Wr - Wmin;

          dJdb = -2 * Error_max * dwdb + 2 * p * beta_old * TL^2;

          beta_new = beta_old - 0.000072*dJdb;                              % 如果不做软切换，学习率必须很小很小,0.3倍时可以设置到0.000068，

          if (beta_new < 0)
              beta_new = 0;
          end

          if (beta_new > 1.0)
              beta_new = 1.0;
          end

      elseif (Wm - Wm_Last > 0.0)
          beta_new = beta_old;

          if (beta_new < 0)
              beta_new = 0;
          end

          if (beta_new > 1.0)
              beta_new = 1.0;
          end
      end

  end

  % 状态3，输出ISE，相关标志位重置
  if (run_flag == 3)
      ISE_Output = error_squa * 0.1;                      % 适当放大一下计算值
      Time_Output = Zero_Crossing_Time;

      % 一次相邻过零点结束，根据过零时间间隔、ISE计算值判断模态
      if (Time_Output > Fd_time_low && Time_Output < Fd_time_Up)
          if (ISE_Output > Fd_ISE)
              Fd_Flag = 1;
          end
      elseif (Time_Output > Fo_time_low && Time_Output < Fo_time_Up)
          if (ISE_Output > Fo_ISE)
              Fo_Flag = 1;
          end
      end

      Zero_Crossing_Time = 0;
      error_squa = 0;

      % 完成一次相邻过零点计算，标志位置零
      run_flag = 0;
      % 完成一次相邻过零点，计数一次
      zero_count = zero_count + 1;
  end

  % 过零情况
  % 第一次完整过零，转速下降
  if (zero_count == 1)
      ISE1 = ISE_Output;
  end
  % 计算了一次ISE以后，开始计算误差为0的时间，如果长期没有下一次，说明当前alpha没有超调，直接置0标志位，不计算ISE2
  if (zeroerr_time >= 50)    % 等待0.001s.10个步长
      ISE2 = 0;
      zero_count = 0;
      zeroerr_time = 0;
  end
  % 第二次完整过零，有超调
  if (zero_count == 2)
      ISE2 = ISE_Output;
      zero_count = 0;
      zeroerr_time = 0;
  end

end


time = time + T;
zero_time = zero_time + T;
errorlast_flag = error_flag;
Wm_Last = Wm;
beta_old = beta_new;

% 相关数据输出
yb1 = error_squa;                                         % 误差平方值，从过零开始一直计算，过零结束清零
yb2 = run_flag;                                           % 状态机标志位
yb3 = ISE_Output;                                         % ISE输出值，一个过零周期结束输出一次
yb4 = ISE1;                                               % 转速下降引起的ISE1
yb5 = ISE2;                                               % 转速超调引起的ISE2
yb6 = Fo_Flag;                                            % 谐振检测标志位，置1代表为谐振
yb7 = Fd_Flag;                                            % 扰动检测标志位，置1代表为扰动出
yb8 = beta_new;

== matlab function Model/MATLAB Function6 ==
  settings: updateMethod=DISCRETE  sampleTime=0.0001
  data: e input; ISE_T output
function ISE_T = calculate_ISE(e)

persistent T time M SumErr SumISE

if isempty(T)
    T = 0.0001;
    time = 0;
    SumErr = 0;
    SumISE = 0;
    M = 0;
end

if (time >= 1)

    SumErr = SumErr + e^2 * T;
    M = M + 1;
    
    % 计算周期为0.01，100个仿真步长
    if (M == 100)
        % 低通滤波，取70%当前值和30%的历史值
        SumISE = SumErr*0.7 + SumISE*0.3;
        SumErr = 0;
        M = 0;
    end

end

time = time + T;

% 最终结果保留三位小数，保留小数的操作主要是为了不要让数值抖动太大
ISE_T = round(SumISE*1000)/1000;

end
